simulink model "DynamicsSolver"  (R2022a)
settings: Solver=VariableStepAuto  StartTime=0.0  StopTime=10.0  RelTol=1e-3
undefined symbols (not defined in the file): CM, CT, d, sqrt22, Tm
libraries: shared6dof x1
settings Model: Creator=Lenovo  LastModifiedBy=Lenovo

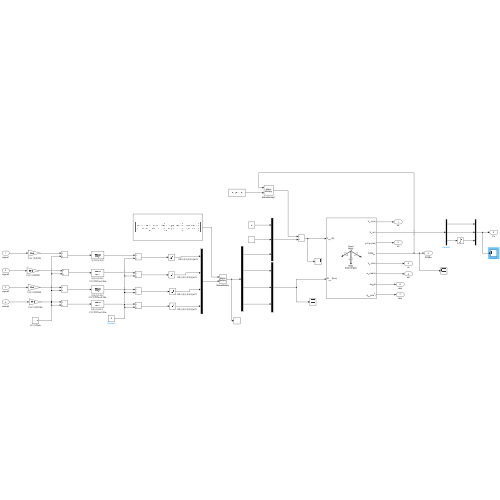
[thumbnail: Simulink's stored preview of the top-level diagram]
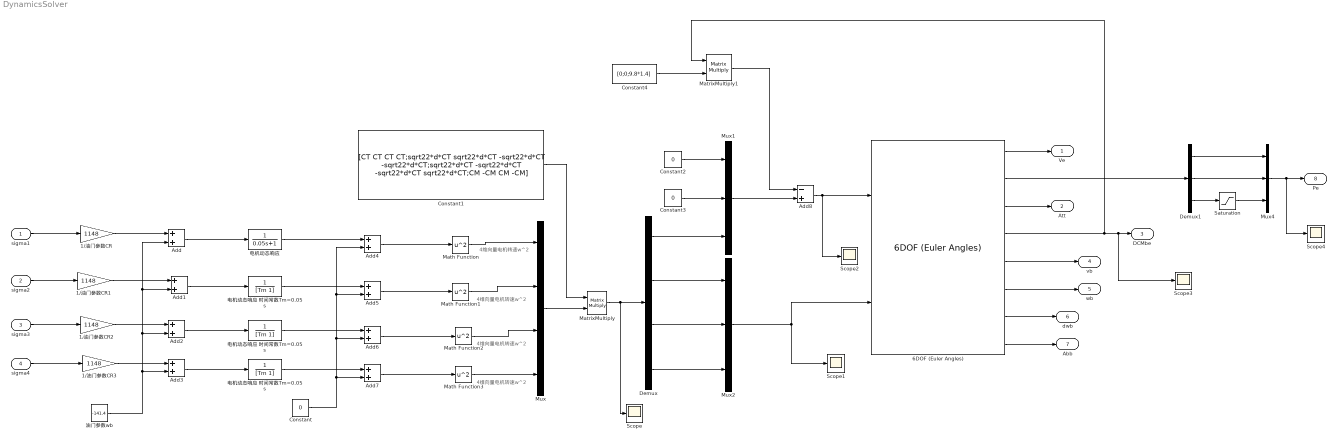
== system DynamicsSolver ==
  note: 4维向量电机转速w^2
  note: 4维向量电机转速w^2
  note: 4维向量电机转速w^2
  note: 4维向量电机转速w^2
  sigma1 : Inport
  sigma2 : Inport  Port=2
  sigma3 : Inport  Port=3
  sigma4 : Inport  Port=4
  1/油门参数CR{,1..3} (4 alike) : Gain  Gain=1148
  6DOF (Euler Angles) : shared6dof/6DOF (Euler Angles)  units=Metric (MKS)  mtype=Fixed  rep=Euler Angles  xme_0=[0 0 0]  Vm_0=[0 0 0]  eul_0=[0 0 0]  pm_0=[0 0 0]  mass_0=1.4  mass_e=0.5  mass_f=2.0  inertia=[0.0211,0,0;0,0.0219,0;0,0,0.0366]  inertia_e=eye(3)  inertia_f=2*eye(3)  k_quat=1.0  vre_flag=on  abi_flag=off  aMode=0  xme_statename=''  Vm_statename=''  eul_statename=''  quat_statename=''  pm_statename=''  mass_statename=''
      settings: SourceProductBaseCode=AE,PW,DR,MT,VE
  Add{,1..7} (8 alike) : Sum
  Add8 : Sum  Inputs=-+
  Constant : Constant  Value=0
  Constant1 : Constant  Value=[CT CT CT CT;sqrt22*d*CT sqrt22*d*CT -sqrt22*d*CT -sqrt22*d*CT;sqrt22*d*CT -sqrt22*d*CT -sqrt22*d*CT sqrt22*d*CT;CM -CM CM -CM]
  Constant2 : Constant  Value=0
  Constant3 : Constant  Value=0
  Constant4 : Constant  Value=[0;0;9.8*1.4]
  Demux : Demux
  Demux1 : Demux  Outputs=3
  Math Function{,1..3} (4 alike) : Math  Operator=square
  MatrixMultiply : Product  Multiplication=Matrix(*)
  MatrixMultiply1 : Product  Multiplication=Matrix(*)
  Mux : Mux
  Mux1 : Mux  Inputs=3
  Mux2 : Mux  Inputs=3
  Mux4 : Mux  Inputs=3
  Saturation : Saturate
  Scope{,1..4} (5 alike) : Scope
  油门参数wb : Constant  Value=-141.4
  电机动态响应 : TransferFcn  Denominator=[0.05 1]
  电机动态响应 时间常数Tm=0.05s : TransferFcn  Denominator=[Tm 1]
  "电机动态响应 时间常数Tm=0.05s " : TransferFcn  Denominator=[Tm 1]
  电机动态响应 时间常数Tm=0.05s : TransferFcn  Denominator=[Tm 1]
  Ve : Outport
  Att : Outport  Port=2
  DCMbe : Outport  Port=3
  vb : Outport  Port=4
  wb : Outport  Port=5
  dwb : Outport  Port=6
  Abb : Outport  Port=7
  Pe : Outport  Port=8
  wires:
  sigma1/1 -> 1/油门参数CR/1
  sigma2/1 -> 1/油门参数CR1/1
  sigma3/1 -> 1/油门参数CR2/1
  sigma4/1 -> 1/油门参数CR3/1
  1/油门参数CR/1 -> Add/1
  1/油门参数CR1/1 -> Add1/1
  1/油门参数CR2/1 -> Add2/1
  1/油门参数CR3/1 -> Add3/1
  油门参数wb/1 -> Add3/2, Add2/2, Add1/2, Add/2
  Add/1 -> 电机动态响应/1
  Add1/1 -> 电机动态响应 时间常数Tm=0.05s/1
  Add2/1 -> "电机动态响应 时间常数Tm=0.05s "/1
  Add3/1 -> 电机动态响应 时间常数Tm=0.05s/1
  电机动态响应/1 -> Add4/1
  电机动态响应 时间常数Tm=0.05s/1 -> Add5/1
  "电机动态响应 时间常数Tm=0.05s "/1 -> Add6/1
  电机动态响应 时间常数Tm=0.05s/1 -> Add7/1
  Constant/1 -> Add7/2, Add6/2, Add5/2, Add4/2
  Add4/1 -> Math Function/1
  Add5/1 -> Math Function1/1
  Add6/1 -> Math Function2/1
  Add7/1 -> Math Function3/1
  Math Function/1 -> Mux/1
  Math Function1/1 -> Mux/2
  Math Function2/1 -> Mux/3
  Math Function3/1 -> Mux/4
  Mux/1 -> MatrixMultiply/2
  Constant1/1 -> MatrixMultiply/1
  MatrixMultiply/1 -> Scope/1, Demux/1
  Demux/2 -> Mux2/1
  Demux/3 -> Mux2/2
  Demux/4 -> Mux2/3
  Demux/1 -> Mux1/3
  Constant2/1 -> Mux1/1
  Constant3/1 -> Mux1/2
  Mux1/1 -> Add8/2
  Add8/1 -> Scope2/1, 6DOF (Euler Angles)/1
  Mux2/1 -> 6DOF (Euler Angles)/2, Scope1/1
  Constant4/1 -> MatrixMultiply1/2
  MatrixMultiply1/1 -> Add8/1
  6DOF (Euler Angles)/1 -> Ve/1
  6DOF (Euler Angles)/8 -> Abb/1
  6DOF (Euler Angles)/7 -> dwb/1
  6DOF (Euler Angles)/6 -> wb/1
  6DOF (Euler Angles)/5 -> vb/1
  6DOF (Euler Angles)/4 -> MatrixMultiply1/1, Scope3/1, DCMbe/1
  6DOF (Euler Angles)/3 -> Att/1
  Mux4/1 -> Scope4/1, Pe/1
  Demux1/2 -> Mux4/2
  Saturation/1 -> Mux4/3
  Demux1/3 -> Saturation/1
  6DOF (Euler Angles)/2 -> Demux1/1
  Demux1/1 -> Mux4/1
